simulink model "connect_sim2"  (R2014a)
settings: Solver=ode45  StartTime=0.0  StopTime=2  FixedStep=1/10000  MaxStep=1e-4  MinStep=1e-4  RelTol=1e-3
settings Model: Creator=Think127  LastModifiedBy=Think127
settings DebuggingCC: UnderspecifiedInitializationDetection=Classic  StateNameClashWarn=warning

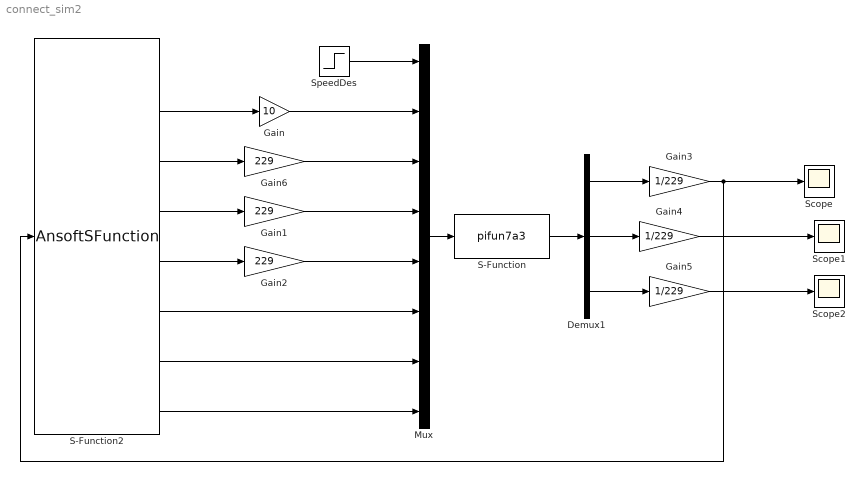
== system connect_sim2 ==
  Demux1 : Demux  Outputs=3
  Gain : Gain  Gain=10
  Gain1 : Gain  Gain=229
  Gain2 : Gain  Gain=229
  Gain3 : Gain  Gain=1/229
  Gain4 : Gain  Gain=1/229
  Gain5 : Gain  Gain=1/229
  Gain6 : Gain  Gain=229
  Mux : Mux  Inputs=8
  S-Function : S-Function  FunctionName=pifun7a3  EnableBusSupport=off
  S-Function2 : S-Function  FunctionName=AnsoftSFunction  EnableBusSupport=off
      settings: OpenFcn=AnsoftLinkDialog();
  Scope : Scope
      settings: TimeRange=2  YMin=0.906  YMax=0.919
  Scope1 : Scope
  Scope2 : Scope
      settings: SaveName=ScopeData2
  SpeedDes : Step  Before=6000  After=0  SampleTime=1/10000
  wires:
  Demux1/1 -> Gain3/1
  Demux1/2 -> Gain4/1
  SpeedDes/1 -> Mux/1
  Mux/1 -> S-Function/1
  S-Function2/2 -> Gain/1
  S-Function2/3 -> Gain6/1
  S-Function2/4 -> Gain1/1
  S-Function2/5 -> Gain2/1
  S-Function2/6 -> Mux/6
  S-Function2/7 -> Mux/7
  S-Function2/8 -> Mux/8
  Gain/1 -> Mux/2
  Gain6/1 -> Mux/3
  Gain2/1 -> Mux/5
  Gain1/1 -> Mux/4
  Gain3/1 -> S-Function2/1, Scope/1
  S-Function/1 -> Demux1/1
  Gain4/1 -> Scope1/1
  Demux1/3 -> Gain5/1
  Gain5/1 -> Scope2/1
